simulink model "task4"  (R2025b)
settings: Solver=VariableStepAuto  StartTime=0.0  StopTime=10.0  MaxStep=0.001  RelTol=1e-3
settings Model: Creator=Администратор  LastModifiedBy=Администратор

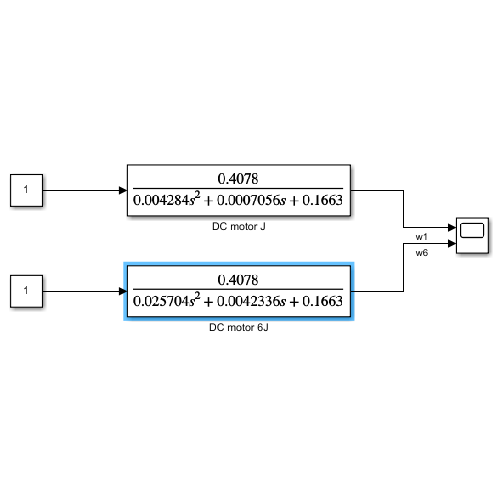
[thumbnail: Simulink's stored preview of the top-level diagram]
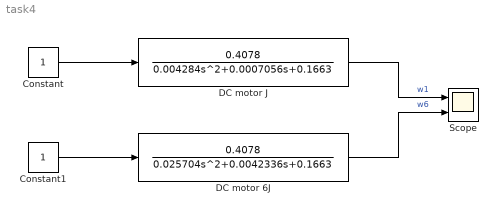
== system task4 ==
  Constant : Constant
  Constant1 : Constant
  DC motor 6J : TransferFcn  Numerator=[0.4078]  Denominator="[0.025704  0.0042336  0.1663]"
  DC motor J : TransferFcn  Numerator=[0.4078]  Denominator="[0.004284  0.0007056  0.1663]"
  Scope : Scope  NumInputPorts=2
      settings: ActiveDisplayYMinimum=-0.60057989741705964  ActiveDisplayYMaximum=5.4052190767535375
  wires:
  Constant/1 -> DC motor J/1
  DC motor J/1 -> Scope/1  "w1"
  Constant1/1 -> DC motor 6J/1
  DC motor 6J/1 -> Scope/2  "w6"
